simulink model "prob2_b"  (R2013a)
settings: Solver=ode45  StartTime=0.0  StopTime=0.0002  RelTol=1e-3
libraries: fl_lib x10, nesl_utility x3, simulink x1, dspswit3 x1
settings Model: Creator=Suddenlink  LastModifiedBy=Suddenlink

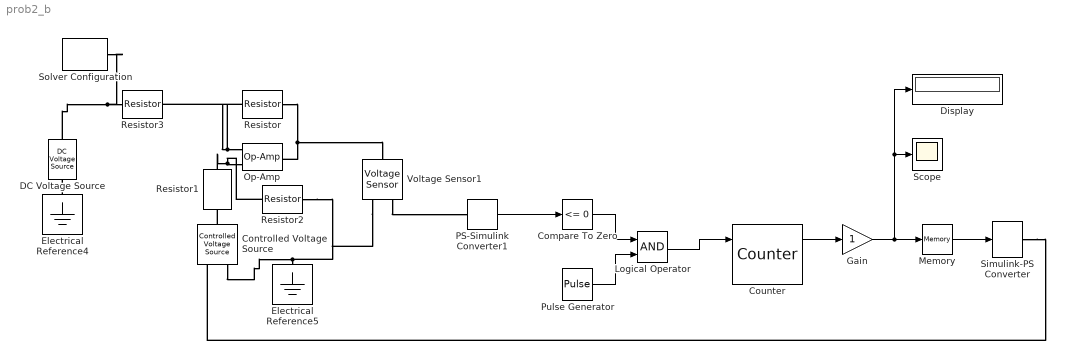
== system prob2_b ==
  Compare To Zero : simulink/Logic and Bit Operations/Compare To Zero  relop=<=  OutDataTypeStr=boolean
  Controlled Voltage Source : fl_lib/Electrical/Electrical Sources/Controlled Voltage Source  i_Log=off  v_Log=off  LocalVarNames=|i|v  LocalVarDescs=|i|v  LocalVarLogging=[0 0]
  Counter : dspswit3/Counter  Direction=Up  CountEvent=Rising edge  CounterSize=User defined  MaxCount=2^4  InitialCount=0  Output=Count and Hit  HitValue=32  ResetInput=on  SamplesPerFrame=1  Ts=1  CntDtype=double  HitDtype=Logical
  DC Voltage Source : fl_lib/Electrical/Electrical Sources/DC Voltage Source  v0=3.1 V  i_Log=off  v_Log=off  LocalVarNames=|i|v  LocalVarDescs=|i|v  LocalVarLogging=[0 0]
  Display : Display
  Electrical Reference4 : fl_lib/Electrical/Electrical Elements/Electrical Reference  i_Log=off  LocalVarNames=|i  LocalVarDescs=|i  LocalVarLogging=0
  Electrical Reference5 : fl_lib/Electrical/Electrical Elements/Electrical Reference  i_Log=off  LocalVarNames=|i  LocalVarDescs=|i  LocalVarLogging=0
  Gain : Gain
  Logical Operator : Logic  AllPortsSameDT=off  OutDataTypeStr=boolean
  Memory : Memory
  Op-Amp : fl_lib/Electrical/Electrical Elements/Op-Amp  i1_Log=off  v1_Log=off  outI_Log=off  LocalVarNames=|i1|v1|outI  LocalVarDescs=|i1|v1|outI  LocalVarLogging=[0 0 0]
  PS-Simulink Converter1 : nesl_utility/PS-Simulink Converter  PhysicalDomain=network_engine_domain  SubClassName=ps_output  LeftPortType=input  RightPortType=output  PseudoPeriodic=off  Frequencies=[]  Unit=1  AffineConversion=off
  Pulse Generator : DiscretePulseGenerator  PulseType=Time based  Period=5e-6  PulseWidth=50
  Resistor{,1..3} (4 alike) : fl_lib/Electrical/Electrical Elements/Resistor  R=1 Ohm  i_Log=off  v_Log=off  LocalVarNames=|i|v  LocalVarDescs=|i|v  LocalVarLogging=[0 0]
  Scope : Scope
      settings: YMin=7  YMax=7
  Simulink-PS Converter : nesl_utility/Simulink-PS Converter  PhysicalDomain=network_engine_domain  SubClassName=ps_input  LeftPortType=input  RightPortType=output  PseudoPeriodic=off  Frequencies=[]  NoiseDistribution=none  NoiseParameters=[]  Unit=1  AffineConversion=off  InputFiltering=off  SimscapeFilterOrder=1  InputFilterTimeConstant=0.001  UdotUserProvided=1
  Solver Configuration : nesl_utility/Solver Configuration  PhysicalDomain=network_engine_domain  SubClassName=solver  LeftPortType=input  RightPortType=generic  Accelerate=off  Tones=[]  Harmonics=[]  SimulateNoise=off  Profile=off  UseLocalSampling=off  EnableSwitchedLinearOptims=on  FrequencyDomain=off  UseCCode=off  UseNewInitialization=off  DoDC=off  ResidualTolerance=1e-09  UseLocalSolver=off  LocalSolverChoice=NE_BACKWARD_EULER_ADVANCER  LocalSolverSampleTime=0.001  DoFixedCost=off  MaxNonlinIter=3  MaxModeIter=2  LinearAlgebra=Sparse  DelaysMemoryBudget=1024
  Voltage Sensor1 : fl_lib/Electrical/Electrical Sensors/Voltage Sensor  i1_Log=off  v1_Log=off  LocalVarNames=|i1|v1  LocalVarDescs=|i1|v1  LocalVarLogging=[0 0]
  wires:
  PS-Simulink Converter1/1 -> Compare To Zero/1
  Compare To Zero/1 -> Logical Operator/1
  Pulse Generator/1 -> Logical Operator/2
  Logical Operator/1 -> Counter/1
  Counter/1 -> Gain/1
  Gain/1 -> Display/1, Scope/1, Memory/1
  Memory/1 -> Simulink-PS Converter/1
  connections:
  Resistor/RConn1 -- Voltage Sensor1/LConn1 -- Op-Amp/RConn1
  Op-Amp/LConn2 -- Resistor3/RConn1 -- Resistor/LConn1
  Voltage Sensor1/RConn1 -- PS-Simulink Converter1/LConn1
  Electrical Reference4/LConn1 -- DC Voltage Source/RConn1
  DC Voltage Source/LConn1 -- Solver Configuration/RConn1 -- Resistor3/LConn1
  Controlled Voltage Source/LConn1 -- Resistor1/RConn1
  Resistor1/LConn1 -- Op-Amp/LConn1 -- Resistor2/LConn1
  Controlled Voltage Source/RConn2 -- Voltage Sensor1/RConn2 -- Resistor2/RConn1 -- Electrical Reference5/LConn1
  Simulink-PS Converter/RConn1 -- Controlled Voltage Source/RConn1
